simulink model "model1"  (R2014a)
settings: Solver=ode45  StartTime=0.0  StopTime=3  RelTol=1e-3
values from neighbouring files (symbols this model uses):
  C9r = [2*(c2V+c2H+c3) c3*(ls+ar) 2*(c2H*l2H-c2V*l2V)+c3*(l3H-l3V) -c2V -c2V -c2H -c2H -c3 -c3;     c3*(ls+ar) 0.5*(c2V+c2H)*s^2+c3*(ls^2+ar^2) c3*(ar*l3H-ls*l3V) -0.5*c2V*s 0.5*c2V*s -0.5*c2H*s 0.5*c2H*s -c3*ls -c3*ar;     2*(c2H*l2H-c2V*l2V)+c3*(l3H-l3V) c3*(ar*l3H-ls*l3V) 2*(c2V*l2V^2+c2H*l2H^2)+c3*(l3V^2+l3H^2) c2V*l2V c2V*l2V -c2H*l2H -c2H*l2H c3*l3V -c3*l3H;     -c2V -0.5*c2V*s c2V*l2V c2V 0 0 0 0  ...(+204 chars)    [data.m]
  h = [0 0 H H 0 0]    [responsetoblock.m]    (also in responsetomultiu.m; successiveblock.m = [h h h h h 0])
  K9r = [2*(k2V+k2H+k3) k3*(ls+ar) 2*(k2H*l2H-k2V*l2V)+k3*(l3H-l3V) -k2V -k2V -k2H -k2H -k3 -k3;     k3*(ls+ar) 0.5*(k2V+k2H)*s^2+k3*(ls^2+ar^2) k3*(ar*l3H-ls*l3V) -0.5*k2V*s 0.5*k2V*s -0.5*k2H*s 0.5*k2H*s -k3*ls -k3*ar;     2*(k2H*l2H-k2V*l2V)+k3*(l3H-l3V) k3*(ar*l3H-ls*l3V) 2*(k2V*l2V^2+k2H*l2H^2)+k3*(l3V^2+l3H^2) k2V*l2V k2V*l2V -k2H*l2H -k2H*l2H k3*l3V -k3*l3H;     -k2V -0.5*k2V*s k2V*l2V k1V+k2V 0 0  ...(+220 chars)    [data.m]
  Kt = [0 0 0 0;     0 0 0 0;     0 0 0 0;     k1V 0 0 0;     0 k1V 0 0;     0 0 k1H 0;     0 0 0 k1H;     0 0 0 0;     0 0 0 0]    [responsetoblock.m]    (also in responsetomultiu.m; successiveblock.m)
  M9 = [m2 0 0 0 0 0 0 0 0;     0 J2x 0 0 0 0 0 0 0;     0 0 J2y 0 0 0 0 0 0;     0 0 0 m1V 0 0 0 0 0;     0 0 0 0 m1V 0 0 0 0;     0 0 0 0 0 m1H 0 0 0;     0 0 0 0 0 0 m1H 0 0;     0 0 0 0 0 0 0 m3 0;     0 0 0 0 0 0 0 0 m3]    [data.m]
  tH = [0 l2/u (l2+H)/u (l2+H+L)/u (l2+2*H+L)/u 30/u]    [responsetoblock.m]    (also in responsetomultiu.m; successiveblock.m = [tH tH(1,20)+s/u+tadd 30/u])
  tV = [0 0 H/u (H+L)/u (2*H+L)/u 30/u]    [responsetoblock.m]    (also in responsetomultiu.m; successiveblock.m = [tV tV(1,20)+s/u+tadd 30/u])
settings Model: Creator=Charlie Ren  LastModifiedBy=Charlie Ren

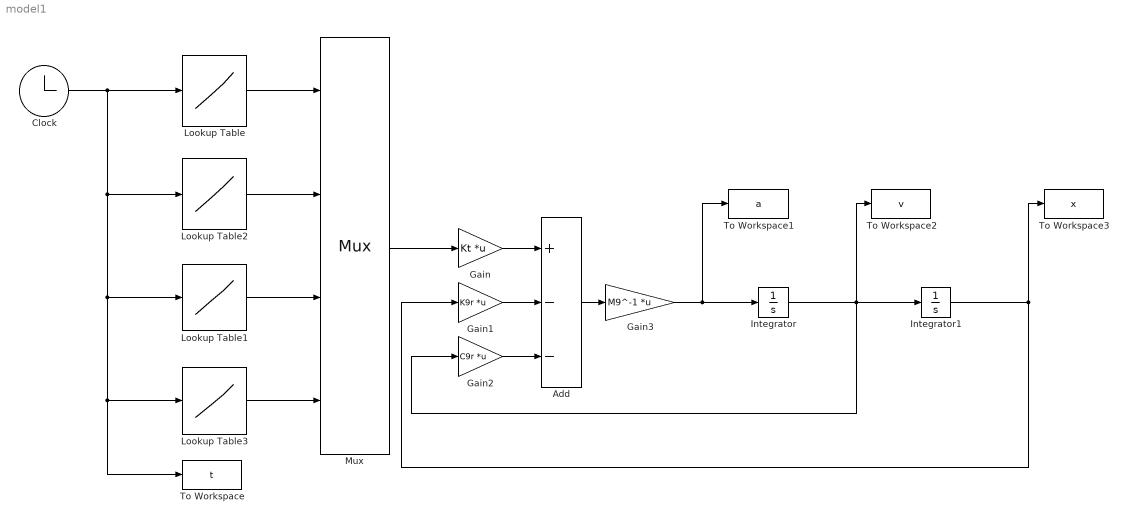
== system model1 ==
  Add : Sum  Inputs=+--
  Clock : Clock
  Gain : Gain  Gain=Kt  Multiplication=Matrix(K*u)
  Gain1 : Gain  Gain=K9r  Multiplication=Matrix(K*u)
  Gain2 : Gain  Gain=C9r  Multiplication=Matrix(K*u)
  Gain3 : Gain  Gain=M9^-1  Multiplication=Matrix(K*u)
  Integrator : Integrator
  Integrator1 : Integrator
  Lookup Table : Lookup  DialogController=Simulink.DDGSource  InputValues=tV  Table=h
  Lookup Table1 : Lookup  DialogController=Simulink.DDGSource  InputValues=tH  Table=h
  Lookup Table2 : Lookup  DialogController=Simulink.DDGSource  InputValues=tV  Table=h
  Lookup Table3 : Lookup  DialogController=Simulink.DDGSource  InputValues=tH  Table=h
  Mux : Mux
  To Workspace : ToWorkspace  VariableName=t  SampleTime=-1
  To Workspace1 : ToWorkspace  VariableName=a  SampleTime=-1
  To Workspace2 : ToWorkspace  VariableName=v  SampleTime=-1
  To Workspace3 : ToWorkspace  VariableName=x  SampleTime=-1
  wires:
  Clock/1 -> Lookup Table2/1, To Workspace/1, Lookup Table3/1, Lookup Table1/1, Lookup Table/1
  Lookup Table/1 -> Mux/1
  Lookup Table1/1 -> Mux/3
  Mux/1 -> Gain/1
  Gain/1 -> Add/1
  Gain1/1 -> Add/2
  Gain2/1 -> Add/3
  Add/1 -> Gain3/1
  Gain3/1 -> To Workspace1/1, Integrator/1
  Integrator/1 -> Gain2/1, Integrator1/1, To Workspace2/1
  Integrator1/1 -> Gain1/1, To Workspace3/1
  Lookup Table2/1 -> Mux/2
  Lookup Table3/1 -> Mux/4
